simulink model "knocksensor"  (R2023b)
settings: Solver=FixedStepAuto  StartTime=0.0  StopTime=5  FixedStep=0.01  MinStep=6.5e-5  RelTol=1e-3
undefined symbols (not defined in the file or in its folder): fdesignblkfcn, gcbh
libraries: dspsigops x1, simulink x1
settings Model: Creator=ASharykin  LastModifiedBy=ASharykin

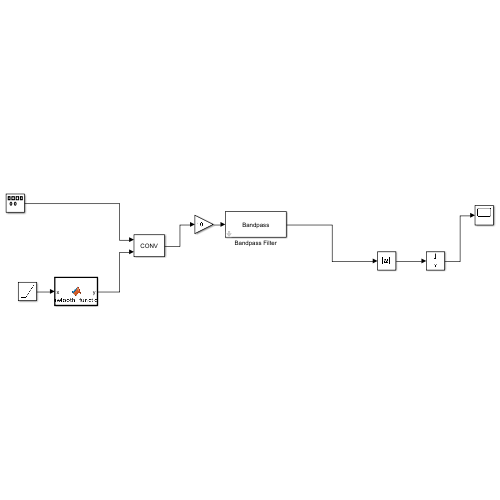
[thumbnail: Simulink's stored preview of the top-level diagram]
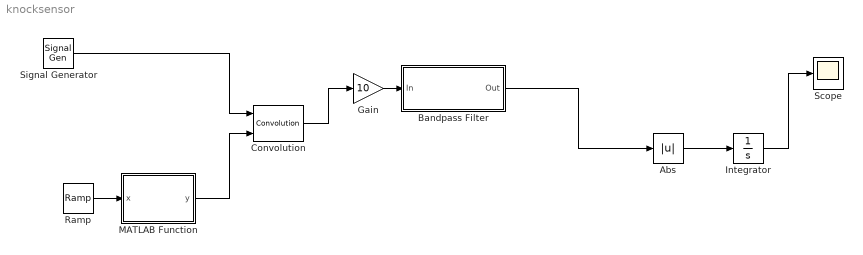
== system knocksensor ==
  Abs : Abs  SaturateOnIntegerOverflow=off
  Bandpass Filter : Subsystem  DialogController=fdesignblkfcn  InitFcn=fdesignblkfcn(gcbh, {'InitFcn'});  mask(Bandpass Filter){}
      mask help: dsp:DSPFilterDesignBlockDialog:BandpassFdesign_MaskDesc
      settings: CopyFcn=fdesignblkfcn(gcbh, {'CopyFcn'});
      mask Help: helpview(mapfilelocation('dsp'), 'dspbandpassfilter');
      mask Display: disp('Bandpass');
  Convolution : dspsigops/Convolution  domain=Time  roundingMode=Floor  overflowMode=off  outputDataTypeStr=Inherit: Same as accumulator  outputMin=[]  outputMax=[]  outputLastDataTypeStr=Inherit: Same as accumulator
  Gain : Gain  Gain=10
  Integrator : Integrator
  MATLAB Function : MATLAB Function  TreatAsAtomicUnit=on
  Ramp : simulink/Sources/Ramp  slope=1  start=0  InitialOutput=0
  Scope : Scope
  Signal Generator : SignalGenerator  Frequency=5000
  wires:
  Signal Generator/1 -> Convolution/1
  Ramp/1 -> MATLAB Function/1(x)
  MATLAB Function/1(y) -> Convolution/2
  Convolution/1 -> Gain/1
  Gain/1 -> Bandpass Filter/1(In)
  Abs/1 -> Integrator/1
  Bandpass Filter/1(Out) -> Abs/1
  Integrator/1 -> Scope/1

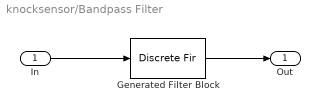
== system knocksensor/Bandpass Filter ==
  In : Inport
  Generated Filter Block : DiscreteFir  Tag=BlockMethodSubSystem  Coefficients=[0.000589704883586056349 -0.000254802803497519107 -0.000207208920154597549 -0.000169579085888164416 -0.00013805296549402647 -0.000112079111119821741 -8.93458531695619142e-05 -7.07474126095356416e-05 -5.49534393713553256e-05 -4.32472209943396369e-05 -3.40287858393766105e-05 -2.79799905111136928e-05 -2.2805635047766417e-05 -1.89280814729038144e-05 -1.42520073552158e-05 -1.01275205361405244e-05 -5.472162339712058e-06 -2.89170982578016832e-06 -1.2572872328949717e-06 -3.89771099794269764e-06 -6.48451467983235039e-06 -1.24744194660495172e-05 -1.65129186706908368e-05 -1.70937733080197586e-05 -1.36923316912698724e-05 -6.34365230560603177e-06 5.04551992629620645e-06 1.69001221998303641e-05 2.60812447874193484e-05 2.81215746464458629e-05 2.21340066038319986e-05 7.75998734338270279e-06 -1.09397322710431304e-05 -3.00567288772665784e-05 -4.28943860388749385e-05 -4.57737862017003512e-05 -3.51748158177795549e-05 -1.35107922815071082e-05 1.57883456024624251e-05 4.36046339115980569e-05 6.31473730505421145e-05 6.63462940886194556e-05 5.0996250249605744e-05 1.91116810605273515e-05 -2.16708310182136621e-05 -6.1341601783577635e-05 -8.72421412914387972e-05 -9.13321718463107942e-05 -6.94976313911701031e-05 -2.62608686212089867e-05 2.91450622466574334e-05 8.11995593421093115e-05 0.000115608285043829152 0.000119961832047462097 9.131005216113223e-05 3.39563449075402706e-05 -3.72965825668802918e-05 -0.000104547630657613562 -0.000147458454155074818 -0.00015299132405557892 -0.000115690486858359182 -4.33915141414108066e-05 4.680210558062278e-05 0.000130355595302456603 0.000184054498924700284 0.000189720045095918854 0.000143334335839298381 5.34296208762042018e-05 -5.70663883104967525e-05 -0.000159563842704425274 -0.000223975655341192184 -0.000230750592914625761 -0.000173476645458529931 -6.49809999776452488e-05 6.86805478013047515e-05 0.000190994577365098108 0.000268186720096515196 0.000275210838268651449 0.000206908035088774448 7.71209486859201522e-05 -8.0903709428930431e-05 -0.000225628396778605809 -0.000315590021132003949 -0.000323718349529835705 -0.000242486696464585855 -9.06269924731813387e-05 9.44284047266882778e-05 0.000262421381156306374 0.000366924918518496098 0.000375064254964674847 0.000280841568344970252 0.00010447860752540864 -0.000108459342342434118 -0.000301904873223104802 -0.000420793219286175408 -0.000429883747980268371 -0.000320943174708211622 -0.000119585753885879356 0.00012364755328644699 0.000342952235867245215 0.000477797175979828115 0.000486860081281969529 0.000363333615278092878 0.000134883720650234612 -0.000139027812774965504 -0.000385979928277622032 -0.000536398501880721982 -0.000546217935859928607 -0.000406614700027966821 -0.000151204940632766174 0.000155184382152018089 0.000429671624600857214 0.000596863906077057344 0.00060643365719066796 0.0004512490572987857 0.000167347275707495878 -0.000171160108134223534 -0.000474401872071800678 -0.000657612640748051749 -0.000667739565861358731 -0.000495803299699136232 -0.000183997036574310184 0.000187753879669637835 0.00051891719318472888 0.000718903839012426929 0.000728544456315715488 0.0005406408899349686 0.000200048271909763781 -0.000203762494365467743 -0.000563425411637934995 -0.000779005986870744344 -0.000788908969270019555 -0.000584328837866797705 -0.000216379250423556725 0.000219754151246944395 0.000606315007310143659 0.000837848078259128106 0.000846984866179882005 0.000626995713959348005 0.000231659456809968161 -0.000234653705621996195 -0.000647777641897740353 -0.000893527679632009171 -0.00090263168731642327 -0.000666976980151998957 -0.000246481458537514599 0.000249224463879829878 0.000686306569707357595 0.000946072671827690218 0.000954056008399305341 0.000704488295194140475 0.000259729858470023143 -0.000262191988276318743 -0.00072207002440071561 -0.000993598442623432315 -0.00100119760029739003 -0.00073802130058014774 -0.000272166013451781961 0.000274095408695620665 0.000753279710715991087 0.00103583149902835431 0.00104197553564634097 0.000767523176228492726 0.000282452287204460395 ...(+24445 chars)]  InputProcessing=Columns as channels (frame based)
  Out : Outport  VectorParamsAs1DForOutWhenUnconnected=off
  wires:
  In/1 -> Generated Filter Block/1
  Generated Filter Block/1 -> Out/1

== matlab function knocksensor/MATLAB Function ==
  data: x input; y output
function y = sawtooth_function(x)
    if x >= 0 && x < 2
        y = 0;
    elseif x >= 2 && x <= 4
        y = 4 - x;
    elseif x > 4
        y = 0;
    else
        error('Input x out of range');
    end
end
